simulink model "Fpump"  (R2025b)
settings: Solver=ode1be  StartTime=0.0  StopTime=300  FixedStep=0.01  RelTol=1e-3
settings Model: Creator=peace  LastModifiedBy=peace
settings RTWCC: GPUComputeCapability=3.5

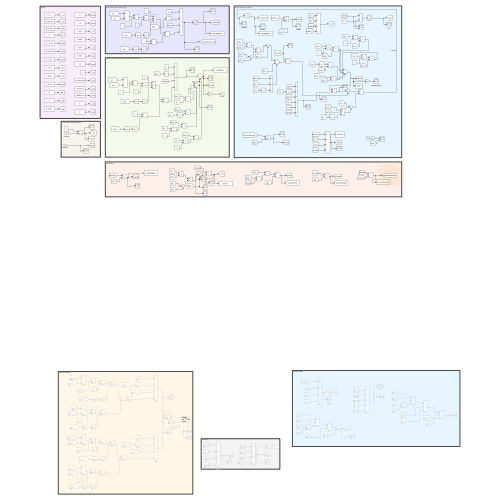
[thumbnail: Simulink's stored preview of the top-level diagram]
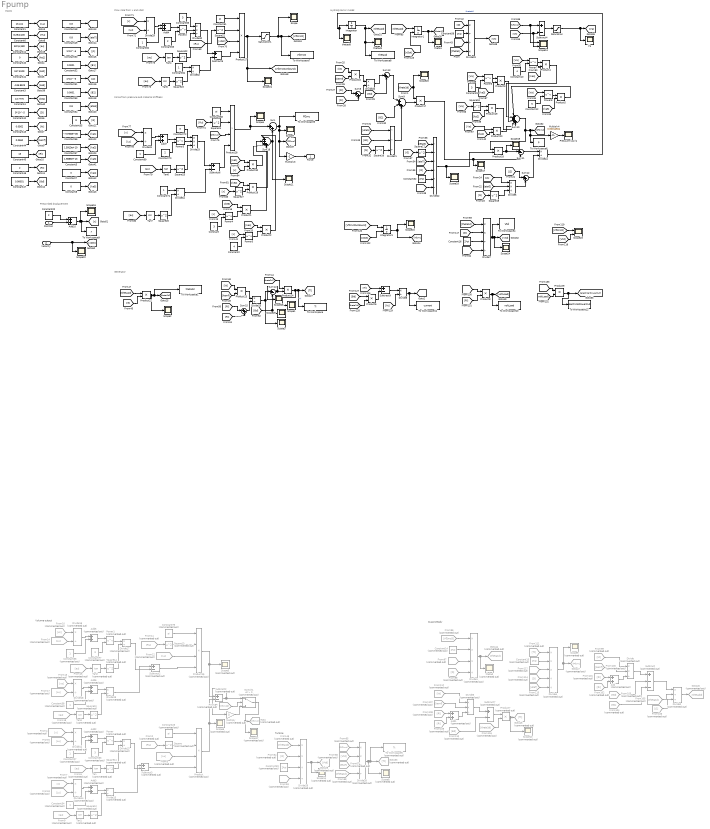
== system Fpump ==
  note: Force from pressure and material stiffness
  note: Flow rate from x and xDot
  note: Turbine
  note: Quasisteady
  note: Generator
  note: Hydrodynamic model
  note: Volume output
  note: Prescribed displacement
  note: Inputs
  Position : Inport
  Velocity : Inport  Port=2
  Add{,1..3,5..6} (6 alike) : Sum  Commented=on
  Add10 : Sum
  Add4 : Sum
  Add7 : Sum
  Constant{,9,65,72} (4 alike) : Constant  Value=3
  Constant1 : Constant  Value=13.411
  Constant10 : Constant  Value=4
  Constant11 : Constant  Value=50*pi/180
  Constant12 : Constant  Value=5
  Constant14 : Constant  Commented=on  Value=2*pi
  Constant15 : Constant  Commented=on  Value=2*pi
  Constant16 : Constant  Value=2*pi
  Constant2 : Constant  Value=4
  Constant{20,46,63,70} (4 alike) : Constant  Value=2
  Constant23 : Constant  Commented=on  Value=pi
  Constant{27,34,36,38} (4 alike) : Constant  Commented=on
  Constant3 : Constant  Value=-135.8523
  Constant32 : Constant  Value=2*pi
  Constant33 : Constant  Commented=on  Value=3
  Constant35 : Constant  Commented=on  Value=pi
  Constant37 : Constant  Commented=on  Value=3
  Constant4 : Constant  Value=13.7775
  Constant40 : Constant  Value=0
  Constant41 : Constant  Value=517.6129
  Constant42 : Constant  Value=5*10^-5
  Constant43 : Constant  Value=0.0562
  Constant44 : Constant  Value=0.0562
  Constant45 : Constant  Value=13
  Constant47 : Constant  Value=0.00001
  Constant48 : Constant  Value=0.8
  Constant49 : Constant  Value=0.8
  Constant5 : Constant  Value=1.9886e+13
  Constant50 : Constant  Value=1*10^-5
  Constant51 : Constant  Value=1*10^-5
  Constant52 : Constant  Value=0.0001
  Constant53 : Constant  Value=0.0001
  Constant54 : Constant  Value=0.8
  Constant55 : Constant  Value=8
  Constant56 : Constant  Value=-7.5786e+06
  Constant57 : Constant  Value=1.5913e+10
  Constant58 : Constant  Value=2*pi
  Constant59 : Constant  Commented=on  Value=2*pi
  Constant6 : Constant  Value=8.29/2/100
  Constant61 : Constant  Value=pi
  Constant{62,64,69,71} (4 alike) : Constant
  Constant68 : Constant  Value=pi
  Constant7 : Constant  Value=0
  Constant8 : Constant  Value=0
  Divide : Product  Commented=on  Inputs=**/
  Divide1 : Product  Commented=on  Inputs=***/
  Divide{11,13..19} (8 alike) : Product  Commented=on  Inputs=*/
  Divide2 : Product  Commented=on  Inputs=*//
  Divide{8,20,24..25,29,31..32,34} (8 alike) : Product  Inputs=*/
  Divide{5,21,30,33} (4 alike) : Product  Inputs=**/
  Divide22 : Product  Inputs=*/**//
  Divide23 : Product  Inputs=*//*
  Divide26 : Product  Commented=on  Inputs=**//
  Divide28 : Product  Commented=on  Inputs=***/
  Divide3 : Product  Commented=on  Inputs=**/
  Divide4 : Product  Commented=on  Inputs=***//
  Divide7 : Product  Inputs=**//
  From10 : From  Commented=on  GotoTag=xs
  From100 : From  Commented=on  GotoTag=kemf
  From101 : From  Commented=on  GotoTag=Rl
  From102 : From  Commented=on  GotoTag=Ri
  From103 : From  Commented=on  GotoTag=Bd
  From104 : From  Commented=on  GotoTag=B1
  From{46,68,105,116} (4 alike) : From  Commented=on  GotoTag=theta1d
  From106 : From  Commented=on  GotoTag=J1
  From107 : From  Commented=on  GotoTag=kemf
  From108 : From  Commented=on  GotoTag=Rl
  From109 : From  Commented=on  GotoTag=Ri
  From11 : From  Commented=on  GotoTag=Ru
  From110 : From  Commented=on  GotoTag=Bd
  From111 : From  Commented=on  GotoTag=Tt
  From112 : From  Commented=on  GotoTag=epsilon
  From113 : From  Commented=on  GotoTag=kt
  From114 : From  Commented=on  GotoTag=D
  From115 : From  Commented=on  GotoTag=etaT
  From{3,5,8,12,14,17} (6 alike) : From  Commented=on  GotoTag=Lu
  From13 : From  Commented=on  GotoTag=xs
  From{6,9,15,18} (4 alike) : From  Commented=on  GotoTag=au
  From2 : From  Commented=on  GotoTag=Ru
  From4 : From  Commented=on  GotoTag=x
  From53 : From  Commented=on  GotoTag=epsilon
  From54 : From  Commented=on  GotoTag=D
  From65 : From  Commented=on  GotoTag=Pf2mc
  From66 : From  Commented=on  GotoTag=Vtd
  From67 : From  Commented=on  GotoTag=etaT
  From7 : From  Commented=on  GotoTag=x
  From89 : From  Commented=on  GotoTag=Vf2mcD
  From96 : From  Commented=on  GotoTag=Vf2mcD
  From97 : From  Commented=on  GotoTag=epsilon
  From98 : From  Commented=on  GotoTag=D
  From99 : From  Commented=on  GotoTag=kt
  Goto : Goto  Commented=on  GotoTag=Vf2mc
  Goto29 : Goto  Commented=on  GotoTag=Vtd
  Goto33 : Goto  Commented=on  GotoTag=Tt
  Goto44 : Goto  Commented=on  GotoTag=theta1d
  Goto45 : Goto  Commented=on  GotoTag=thetadd
  Goto46 : Goto  Commented=on  GotoTag=Tt
  Goto47 : Goto  Commented=on  GotoTag=Pf2mc
  Integrator : Integrator  LowerSaturationLimit=0
  Integrator1 : Integrator  ExternalReset=rising  LowerSaturationLimit=0  ShowStatePort=on
  Integrator3 : Integrator  ExternalReset=rising  LimitOutput=on  LowerSaturationLimit=0
  Multiply : Gain  Commented=on  Gain=0
  Multiply3 : Gain  Gain=-1
  Multiply4 : Gain  Gain=0.00014504
  Power : Math  Commented=on  Operator=pow
  Power1 : Math  Commented=on  Operator=pow
  Power{2..8} (7 alike) : Math  Operator=pow
  Pressure (psi)1 : Scope
      settings: ActiveDisplayYMinimum=-5.2350685226867055  ActiveDisplayYMaximum=46.0529725245055  DataLoggingVariableName=ScopeData31
  Product : Product  Commented=on  Inputs=4
  Product{1..6,8..9,16..20,22..24,29..30} (18 alike) : Product
  Product15 : Product  Commented=on  Inputs=4
  Product27 : Product  Inputs=4
  Product28 : Product  Inputs=4
  Product7 : Product  Commented=on
  Saturation : Saturate  UpperLimit=Inf  LowerLimit=0
  Saturation1 : Saturate  UpperLimit=Inf  LowerLimit=0
  Scope{,1..4,7,11,15..22,24..26} (18 alike) : Scope
      Scope settings: ActiveDisplayYMinimum=-0.0002974405236766963  ActiveDisplayYMaximum=0.0026769647130902669  DataLoggingVariableName=ScopeData9
      Scope1 settings: ActiveDisplayYMinimum=-1  ActiveDisplayYMaximum=1
      Scope11 settings: ActiveDisplayYMinimum=-1  ActiveDisplayYMaximum=1  DataLoggingVariableName=ScopeData22
      Scope15 settings: ActiveDisplayYMinimum=-0.0019537552640037036  ActiveDisplayYMaximum=0.006770628497362245  DataLoggingVariableName=ScopeData23
      Scope16 settings: ActiveDisplayYMinimum=-252.26449603163294  ActiveDisplayYMaximum=32.802699799920319  DataLoggingVariableName=ScopeData16
      Scope17 settings: ActiveDisplayYMinimum=-0.0012501747023492692  ActiveDisplayYMaximum=0.011251572321143424  DataLoggingVariableName=ScopeData24
      Scope18 settings: ActiveDisplayYMinimum=8.9471839432434613E-8  ActiveDisplayYMaximum=1.0947183943243461E-7  DataLoggingVariableName=ScopeData25
      Scope19 settings: ActiveDisplayYMinimum=-1  ActiveDisplayYMaximum=1  DataLoggingVariableName=ScopeData26
      Scope2 settings: ActiveDisplayYMinimum=-1  ActiveDisplayYMaximum=1  DataLoggingVariableName=ScopeData2
      Scope20 settings: ActiveDisplayYMinimum=-1  ActiveDisplayYMaximum=1  DataLoggingVariableName=ScopeData27
      Scope21 settings: ActiveDisplayYMinimum=-0.0029716343329251682  ActiveDisplayYMaximum=0.0029742913341183983  DataLoggingVariableName=ScopeData28
      Scope22 settings: ActiveDisplayYMinimum=-49.848081295924871  ActiveDisplayYMaximum=357.87833617632754  DataLoggingVariableName=ScopeData29
      Scope24 settings: ActiveDisplayYMinimum=-0.00029773600612088347  ActiveDisplayYMaximum=0.0026796240550879518  DataLoggingVariableName=ScopeData8
      Scope25 settings: ActiveDisplayYMinimum=-1  ActiveDisplayYMaximum=1  DataLoggingVariableName=ScopeData18
      Scope26 settings: ActiveDisplayYMinimum=-1  ActiveDisplayYMaximum=1  DataLoggingVariableName=ScopeData30
      Scope3 settings: ActiveDisplayYMinimum=-1  ActiveDisplayYMaximum=1  DataLoggingVariableName=ScopeData15
      Scope4 settings: ActiveDisplayYMinimum=-9.8365616245553262  ActiveDisplayYMaximum=88.529054620997954  DataLoggingVariableName=ScopeData21
      Scope7 settings: ActiveDisplayYMinimum=1511.4943139438367  ActiveDisplayYMaximum=2869.1677360104177  DataLoggingVariableName=ScopeData13
  Scope{5..6,8..10,12,14} (7 alike) : Scope  Commented=on
      Scope10 settings: ActiveDisplayYMinimum=-1  ActiveDisplayYMaximum=1  DataLoggingVariableName=ScopeData20
      Scope12 settings: ActiveDisplayYMinimum=-0.00094087179819930442  ActiveDisplayYMaximum=0.0084678461837937417  DataLoggingVariableName=ScopeData2
      Scope14 settings: ActiveDisplayYMinimum=-4.3E-5  ActiveDisplayYMaximum=4E-5  DataLoggingVariableName=ScopeData4
      Scope5 settings: ActiveDisplayYMinimum=0.07038  ActiveDisplayYMaximum=0.09038  DataLoggingVariableName=ScopeData5
      Scope6 settings: ActiveDisplayYMinimum=0.07191  ActiveDisplayYMaximum=0.08132  DataLoggingVariableName=ScopeData6
      Scope8 settings: ActiveDisplayYMinimum=-0.85985  ActiveDisplayYMaximum=7.73866  DataLoggingVariableName=ScopeData11
      Scope9 settings: ActiveDisplayYMinimum=-31513.593136006442  ActiveDisplayYMaximum=283622.33822405804  DataLoggingVariableName=ScopeData19
  Scope13 : Scope  NumInputPorts=2
      settings: ActiveDisplayYMinimum=-0.00074417995156260907  ActiveDisplayYMaximum=0.0066297811698070768  DataLoggingVariableName=ScopeData7
  Scope23 : Scope  NumInputPorts=2
      settings: ActiveDisplayYMinimum=-0.00060463454147285521  ActiveDisplayYMaximum=0.0016047077017932374  DataLoggingVariableName=ScopeData10
  Square{,11..15} (6 alike) : Math  Commented=on  Operator=square
  Square{16..19,21..27} (11 alike) : Math  Operator=square
  Subtract : Sum  Commented=on  Inputs=+--
  Subtract{1..3,7} (4 alike) : Sum  Commented=on  Inputs=+-
  Subtract{4..6,9} (4 alike) : Sum  Inputs=+-
  Sum{,8,12,15} (4 alike) : Sum  Inputs=|++
  Sum10 : Sum  Inputs=|+++++
  Sum11 : Sum  Inputs=|+-
  Sum13 : Sum  Inputs=|+-
  Sum14 : Sum  Inputs=|+-
  Sum18 : Sum  Inputs=|++++
  Sum9 : Sum  Inputs=|+++
  Switch1 : Switch  Commented=on  Criteria=u2 > Threshold  SaturateOnIntegerOverflow=off  InputSameDT=off
  Tan : Trigonometry  Commented=on  Operator=tan
  Tan1 : Trigonometry  Commented=on
  Tan2 : Trigonometry  Commented=on  Operator=tan
  Tan3 : Trigonometry  Commented=on
  Tan4 : Trigonometry  Operator=tan
  Tan5 : Trigonometry
  Tan6 : Trigonometry  Operator=tan
  Tan7 : Trigonometry
  To Workspace : ToWorkspace  VariableName=Tl  SaveFormat=Timeseries  SampleTime=-1
  To Workspace1 : ToWorkspace  VariableName=theta2d  SaveFormat=Timeseries  SampleTime=-1
  To Workspace10 : ToWorkspace  VariableName=voltLoad  SaveFormat=Timeseries  SampleTime=-1
  To Workspace11 : ToWorkspace  VariableName=current  SaveFormat=Timeseries  SampleTime=-1
  To Workspace12 : ToWorkspace  VariableName=electricalPowerOut  SaveFormat=Timeseries  SampleTime=-1
  To Workspace3 : ToWorkspace  VariableName=Ff2mc  SaveFormat=Timeseries  SampleTime=-1
  To Workspace4 : ToWorkspace  VariableName=Vtd  SaveFormat=Timeseries  SampleTime=-1
  To Workspace5 : ToWorkspace  Commented=on  VariableName=Tt  SampleTime=-1
  To Workspace6 : ToWorkspace  VariableName=P  SaveFormat=Timeseries  SampleTime=-1
  To Workspace7 : ToWorkspace  VariableName=Vf2mcD  SampleTime=-1
  To Workspace8 : ToWorkspace  VariableName=theta1d  SaveFormat=Timeseries  SampleTime=-1
  To Workspace9 : ToWorkspace  VariableName=x  SaveFormat=Timeseries  SampleTime=-1
  Va : Scope
      settings: ActiveDisplayYMinimum=-1.4280417769716719E+8  ActiveDisplayYMaximum=1.2852375992745049E+9  DataLoggingVariableName=ScopeData3
  theta1 : Scope
      settings: ActiveDisplayYMinimum=-159.1776053962563  ActiveDisplayYMaximum=1432.5984485663068  DataLoggingVariableName=ScopeData14
  thetad : Scope  Commented=on
      settings: ActiveDisplayYMinimum=-14.71321151300695  ActiveDisplayYMaximum=21.65771433027281  DataLoggingVariableName=ScopeData17
  thetad1 : Scope
      settings: ActiveDisplayYMinimum=-29.077140697225261  ActiveDisplayYMaximum=255.83472181501602  DataLoggingVariableName=ScopeData12
  thetadd : Scope
      settings: ActiveDisplayYMinimum=-192.46968317119234  ActiveDisplayYMaximum=271.00282624884886
  Force : Outport
  wires:
  Constant11/1 -> [au]
  Constant1/1 -> [Lu]
  Constant6/1 -> [Ru]
  From2/1 -> Square/1
  Constant23/1 -> Product/1
  Square/1 -> Product/2
  From3/1 -> Product/3
  From5/1 -> Divide11/2
  Divide11/1 -> Add2/1
  Constant27/1 -> Add2/2
  Add2/1 -> Power/1
  Constant33/1 -> Power/2
  Power/1 -> Divide13/1
  From6/1 -> Tan/1
  Tan/1 -> Square11/1
  Square11/1 -> Divide13/2
  Tan1/1 -> Square12/1
  From9/1 -> Tan1/1
  Constant34/1 -> Add3/2
  Square12/1 -> Divide15/2
  From8/1 -> Divide14/2
  From7/1 -> Divide14/1
  Add3/1 -> Divide15/1
  Divide14/1 -> Add3/1
  Divide13/1 -> Subtract3/2
  Divide15/1 -> Subtract3/1
  Subtract3/1 -> Product/4
  Tan2/1 -> Square14/1
  Subtract2/1 -> Product15/4
  From15/1 -> Tan2/1
  From10/1 -> Divide16/1
  Divide19/1 -> Subtract2/1
  From14/1 -> Divide16/2
  Divide18/1 -> Add6/1
  From13/1 -> Divide18/1
  From17/1 -> Divide18/2
  Tan3/1 -> Square15/1
  Constant38/1 -> Add6/2
  From18/1 -> Tan3/1
  Constant37/1 -> Power1/2
  Square13/1 -> Product15/2
  Constant36/1 -> Add5/2
  Constant35/1 -> Product15/1
  From11/1 -> Square13/1
  Square14/1 -> Divide17/2
  Power1/1 -> Divide17/1
  Add5/1 -> Power1/1
  Add6/1 -> Divide19/1
  Square15/1 -> Divide19/2
  From12/1 -> Product15/3
  Divide16/1 -> Add5/1
  Product15/1 -> Subtract1/1, Scope5/1
  From4/1 -> Divide11/1
  Divide17/1 -> Subtract2/2
  Product/1 -> Subtract1/2, Scope6/1
  Constant40/1 -> [ke1]
  Constant41/1 -> [ke2]
  Constant42/1 -> [D]
  Constant43/1 -> [kt]
  Constant44/1 -> [kemf]
  Constant46/1 -> [Ri]
  Constant47/1 -> [Bd]
  Constant45/1 -> [Rl]
  Constant48/1 -> [epsilon]
  Constant49/1 -> [etaT]
  Constant50/1 -> [J1]
  Constant52/1 -> [B1]
  Constant51/1 -> [J2]
  Constant53/1 -> [B2]
  Constant54/1 -> [etaG]
  Constant55/1 -> [G]
  [Rl] -> Sum8/1
  [Ri] -> Sum8/2
  [kt] -> Product16/1
  [kemf] -> Product16/2
  Product16/1 -> Divide20/1
  Sum8/1 -> Divide20/2
  Divide20/1 -> Sum13/1
  [Bd] -> Sum13/2
  [B2] -> Sum9/2
  [etaG] -> Divide21/1
  [G] -> Square16/1
  Square16/1 -> Divide21/3
  [B1] -> Divide21/2
  Sum9/1 -> Product17/2
  Square17/1 -> Divide22/2
  [G] -> Square17/1
  [etaG] -> Divide22/1
  [etaT] -> Divide22/3
  [D] -> Divide22/4
  Constant32/1 -> Divide22/5
  [epsilon] -> Divide22/6
  Constant56/1 -> [ka1]
  Constant57/1 -> [ka2]
  Divide22/1 -> Scope18/1, Product18/2
  [D] -> Divide23/1
  [epsilon] -> Divide23/3
  Constant58/1 -> Divide23/2
  Square18/1 -> Product19/1
  [ka2] -> Product19/2
  [ka1] -> Product20/2
  Product19/1 -> Sum10/4
  Product20/1 -> Sum10/5
  Sum10/1 -> To Workspace6/1, Multiply4/1, [Pf2mc], Product18/1
  Product18/1 -> Sum11/1, Scope19/1
  Product17/1 -> Scope17/1, Sum11/2
  Sum11/1 -> Divide24/1
  [J1] -> Divide5/1
  [G] -> Square19/1
  [etaG] -> Divide5/2
  Square19/1 -> Divide5/3
  [J2] -> Sum12/1
  Divide5/1 -> Sum12/2
  Sum12/1 -> Divide24/2
  Divide24/1 -> Integrator/1, thetadd/1  "thetadd"
  [theta1d] -> Product22/1
  [G] -> Product22/2
  Product22/1 -> Scope2/1, To Workspace1/1, [theta2d]
  Sum13/1 -> Sum9/1
  Divide21/1 -> Sum9/3
  [Ri] -> Sum15/2
  Product23/1 -> Divide25/1
  [Rl] -> Sum15/1
  [Bd] -> Scope25/1, Sum14/2
  [kemf] -> Product23/2
  [kt] -> Product23/1
  Divide25/1 -> Sum14/1, Scope3/1
  Sum15/1 -> Divide25/2
  Sum14/1 -> Product24/2, Scope26/1
  Product24/1 -> Scope1/1, To Workspace/1, [Tl]  "Tl"
  [theta2d] -> Product24/1
  From46/1 -> Divide26/1
  From54/1 -> Divide26/2
  Constant59/1 -> Divide26/3
  From53/1 -> Divide26/4
  Divide26/1 -> Scope14/1, Goto29/1
  From65/1 -> Divide28/1
  From66/1 -> Divide28/2
  From67/1 -> Divide28/3
  From68/1 -> Divide28/4
  Divide28/1 -> Scope8/1, To Workspace5/1, Goto33/1
  Tan4/1 -> Square22/1
  Divide32/1 -> Subtract5/2
  [au] -> Tan4/1
  [Lu] -> Divide29/2
  Tan5/1 -> Square23/1
  Square21/1 -> Product27/2
  Constant62/1 -> Add4/2
  Constant64/1 -> Divide32/1
  Divide30/1 -> Subtract5/1
  [au] -> Tan5/1
  Square22/1 -> Divide30/3
  Constant61/1 -> Product27/1
  [Ru] -> Square21/1
  Power2/1 -> Divide30/2
  Add4/1 -> Power2/1
  [xDot] -> Product27/3
  [x] -> Divide29/1
  Constant63/1 -> Power2/2
  Divide29/1 -> Add4/1
  Constant65/1 -> Divide30/1
  Product27/1 -> Saturation1/1, [Vf2mcDUnbound], Scope21/1
  Saturation1/1 -> [Vf2mcD], To Workspace7/1, Scope/1
  [Ru] -> Square24/1
  Constant72/1 -> Divide33/1
  [x] -> Divide31/1
  Add7/1 -> Power3/1
  [au] -> Tan7/1
  Divide31/1 -> Add7/1
  Constant70/1 -> Power3/2
  Constant71/1 -> Divide34/1
  Power3/1 -> Divide33/2
  Square26/1 -> Divide34/2
  [au] -> Tan6/1
  Square25/1 -> Divide33/3
  [Lu] -> Divide31/2
  Divide34/1 -> Subtract6/2
  Tan6/1 -> Square25/1
  Constant69/1 -> Add7/2
  Tan7/1 -> Square26/1
  Divide33/1 -> Subtract6/1
  Constant68/1 -> Product28/1
  Square24/1 -> Product28/2
  [Pf2mc] -> Product28/3
  Subtract6/1 -> Product28/4
  [ke2] -> Product29/1
  [x] -> Square27/1
  Square27/1 -> Product29/2
  [ke1] -> Product30/1
  [x] -> Product30/2
  Product28/1 -> Scope4/1, Sum/1
  Product29/1 -> Sum18/2
  Product30/1 -> Sum18/3
  Subtract5/1 -> Product27/4
  Square23/1 -> Divide32/2
  [Va] -> Square18/1
  [Va] -> Product20/1
  [theta1d] -> Integrator1/1
  Integrator1/1 -> theta1/1, [theta1]
  Divide23/1 -> [Vt]
  Subtract1/1 -> Multiply/1, Switch1/1
  Switch1/1 -> Scope12/1, Goto/1
  From89/1 -> Switch1/2
  Multiply/1 -> Switch1/3
  [Vf2mcDUnbound] -> Integrator3/1
  [theta1d] -> Product17/1, Scope20/1
  [theta1] -> Divide23/4
  Power4/1 -> Product1/2
  [ke3] -> Product1/1
  [x] -> Power4/1
  Constant/1 -> Power4/2
  [x] -> Power5/1
  Power5/1 -> Product2/2
  Constant2/1 -> Power5/2
  [ke4] -> Product2/1
  Constant3/1 -> [ke3]
  Constant4/1 -> [ke4]
  Product1/1 -> Sum18/4
  Constant7/1 -> [ka4]
  Constant5/1 -> [ka3]
  Constant8/1 -> [ka5]
  Product3/1 -> Sum10/3
  [Va] -> Power6/1
  Power6/1 -> Product3/1
  [ka3] -> Product3/2
  Constant9/1 -> Power6/2
  [ka4] -> Product4/2
  Product4/1 -> Sum10/2
  [Va] -> Power7/1
  Constant10/1 -> Power7/2
  Power7/1 -> Product4/1
  Product5/1 -> Sum10/1
  [Va] -> Power8/1
  [ka5] -> Product5/2
  Power8/1 -> Product5/1
  Constant12/1 -> Power8/2
  Integrator/1 -> [theta1d], To Workspace8/1, thetad1/1
  From96/1 -> Divide1/1
  Constant14/1 -> Divide1/2
  From97/1 -> Divide1/3
  From98/1 -> Divide1/4
  Divide1/1 -> thetad/1, Goto44/1
  From101/1 -> Add/1
  From102/1 -> Add/2
  From99/1 -> Divide/1
  From100/1 -> Divide/2
  Add/1 -> Divide/3
  Divide/1 -> Subtract/1
  From103/1 -> Subtract/2
  From104/1 -> Subtract/3
  Subtract/1 -> Divide2/1
  From105/1 -> Divide2/2
  From106/1 -> Divide2/3
  Divide2/1 -> Goto45/1
  Divide3/1 -> Subtract7/1
  From113/1 -> Divide3/1
  From109/1 -> Add1/2
  From107/1 -> Divide3/2
  From108/1 -> Add1/1
  Add1/1 -> Divide3/3
  From110/1 -> Subtract7/2
  Divide4/1 -> Scope9/1, Goto47/1
  Subtract7/1 -> Product7/1
  From116/1 -> Product7/2
  Product7/1 -> Scope10/1, Goto46/1
  From111/1 -> Divide4/1
  From112/1 -> Divide4/3
  Constant15/1 -> Divide4/2
  From114/1 -> Divide4/4
  From115/1 -> Divide4/5
  Product2/1 -> Sum18/1
  Sum18/1 -> Sum/2, Scope11/1
  Sum/1 -> Scope7/1, Multiply3/1, [Ff2mc], To Workspace3/1
  [Vf2mc] -> Scope13/1, Subtract4/1
  Subtract4/1 -> Saturation/1
  Velocity/1 -> Scope22/1, [xDot]
  Add10/1 -> Scope16/1, To Workspace9/1, [x]
  Constant20/1 -> Add10/1
  Position/1 -> Add10/2
  Multiply3/1 -> Force/1
  Multiply4/1 -> Pressure (psi)1/1
  Saturation/1 -> Va/1, [Va]
  [Vt] -> Subtract4/2, Scope13/2
  [xDot] -> Integrator1/2
  Constant16/1 -> Divide7/3
  [epsilon] -> Divide7/4
  Divide7/1 -> [Vtd], Scope24/1, To Workspace4/1
  [theta1d] -> Divide7/1
  [D] -> Divide7/2
  [Vtd] -> Scope23/2
  [Vf2mcD] -> Scope23/1
  Integrator3/1 -> Scope15/1, [Vf2mc]
  [xDot] -> Integrator3/2
  [Bd] -> Product6/1
  [theta2d] -> Product6/2
  [Tl] -> Subtract9/1
  Product6/1 -> Subtract9/2
  Subtract9/1 -> Divide8/1
  [kt] -> Divide8/2
  Divide8/1 -> To Workspace11/1, [current]
  [current] -> Product8/1
  [Rl] -> Product8/2
  Product8/1 -> To Workspace10/1, [voltLoad]
  [current] -> Product9/1
  [voltLoad] -> Product9/2
  Product9/1 -> To Workspace12/1, [electricalPowerOut]
